simulink model "TestModel"  (R2023a)
settings: Solver=VariableStepAuto  StartTime=0.0  StopTime=10.0  RelTol=1e-3
settings Model: Creator=Martin  LastModifiedBy=Martin

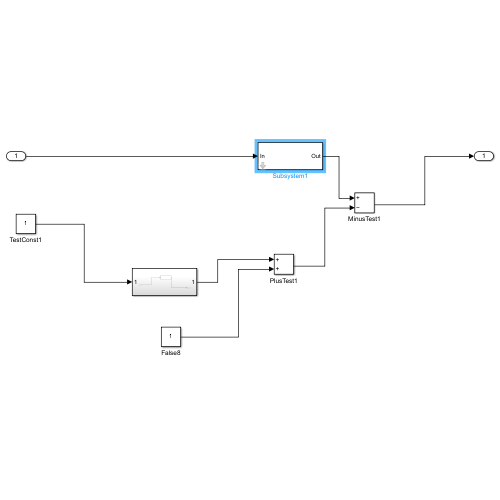
[thumbnail: Simulink's stored preview of the top-level diagram]
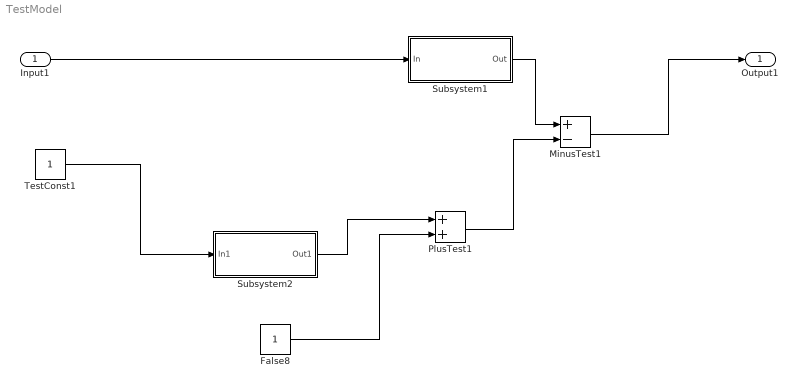
== system TestModel ==
  Input1 : Inport
  False8 : Constant
  MinusTest1 : Sum  Inputs=+-
  PlusTest1 : Sum
  Subsystem1 : Subsystem
  Subsystem2 : Subsystem
  TestConst1 : Constant
  Output1 : Outport
  wires:
  Input1/1 -> Subsystem1/1(In)
  MinusTest1/1 -> Output1/1
  Subsystem2/1(Out1) -> PlusTest1/1
  False8/1 -> PlusTest1/2
  Subsystem1/1(Out) -> MinusTest1/1
  PlusTest1/1 -> MinusTest1/2
  TestConst1/1 -> Subsystem2/1(In1)

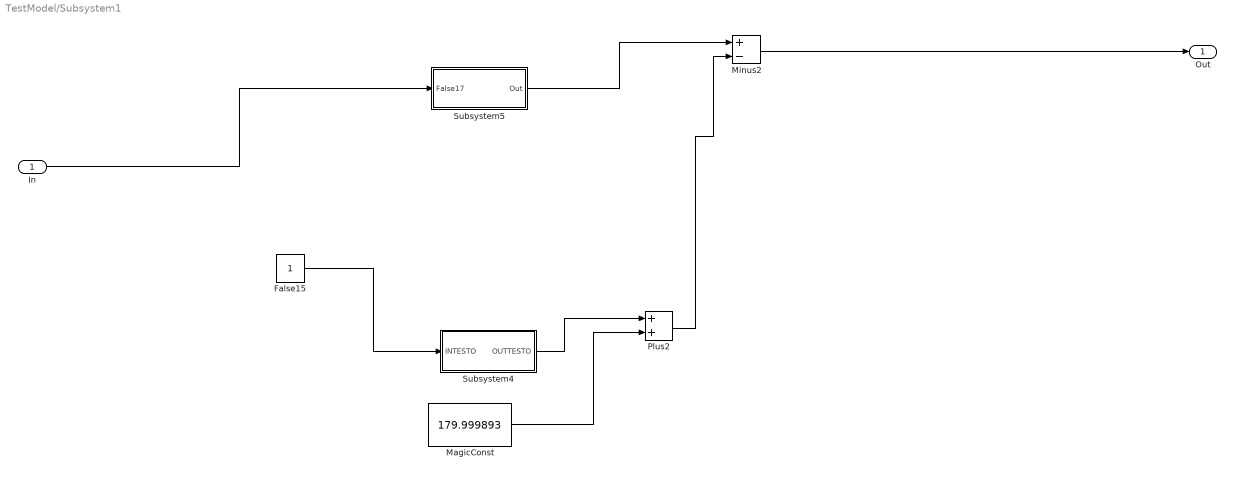
== system TestModel/Subsystem1 ==
  In : Inport
  False15 : Constant
  MagicConst : Constant  Value=179.999893
  Minus2 : Sum  Inputs=+-
  Plus2 : Sum
  Subsystem4 : Subsystem
  Subsystem5 : Subsystem
  Out : Outport
  wires:
  False15/1 -> Subsystem4/1(INTESTO)
  Plus2/1 -> Minus2/2
  MagicConst/1 -> Plus2/2
  Subsystem4/1(OUTTESTO) -> Plus2/1
  Minus2/1 -> Out/1
  Subsystem5/1(Out) -> Minus2/1
  In/1 -> Subsystem5/1(False17)

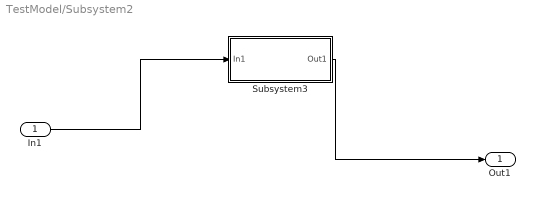
== system TestModel/Subsystem2 ==
  In1 : Inport
  Subsystem3 : Subsystem
  Out1 : Outport
  wires:
  Subsystem3/1(Out1) -> Out1/1
  In1/1 -> Subsystem3/1(In1)

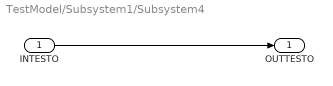
== system TestModel/Subsystem1/Subsystem4 ==
  INTESTO : Inport
  OUTTESTO : Outport
  wires:
  INTESTO/1 -> OUTTESTO/1

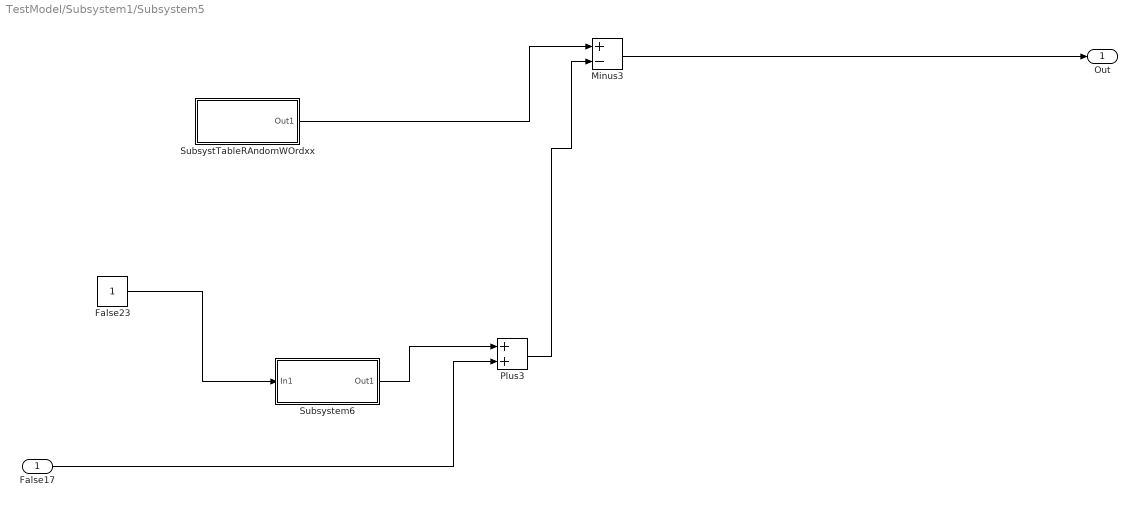
== system TestModel/Subsystem1/Subsystem5 ==
  False17 : Inport
  False23 : Constant
  Minus3 : Sum  Inputs=+-
  Plus3 : Sum
  SubsystTableRAndomWOrdxx : Subsystem
  Subsystem6 : Subsystem
  Out : Outport
  wires:
  SubsystTableRAndomWOrdxx/1(Out1) -> Minus3/1
  Minus3/1 -> Out/1
  Subsystem6/1(Out1) -> Plus3/1
  Plus3/1 -> Minus3/2
  False23/1 -> Subsystem6/1(In1)
  False17/1 -> Plus3/2

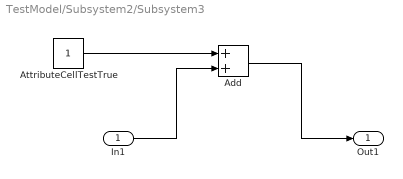
== system TestModel/Subsystem2/Subsystem3 ==
  In1 : Inport
  Add : Sum
  AttributeCellTestTrue : Constant
  Out1 : Outport
  wires:
  Add/1 -> Out1/1
  In1/1 -> Add/2
  AttributeCellTestTrue/1 -> Add/1

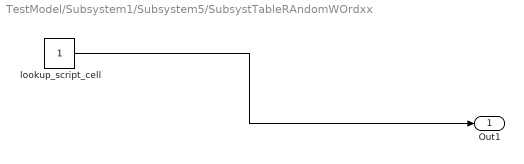
== system TestModel/Subsystem1/Subsystem5/SubsystTableRAndomWOrdxx ==
  lookup_script_cell : Constant
  Out1 : Outport
  wires:
  lookup_script_cell/1 -> Out1/1

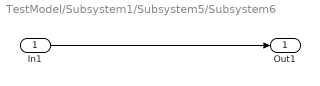
== system TestModel/Subsystem1/Subsystem5/Subsystem6 ==
  In1 : Inport
  Out1 : Outport
  wires:
  In1/1 -> Out1/1
